simulink model "Phase_Estimator_4"  (R2020b)
settings: Solver=ode3  StartTime=0.0  StopTime=t(end)  FixedStep=1/60  RelTol=1e-3  EnableMultiTasking=on
undefined symbols (not defined in the file or in its folder): Activity, gamma_d, gamma_omg, x_initial, zeta
settings Model: Creator=wangf7  LastModifiedBy=chukw
settings DataIOCC: LimitDataPoints=on  SaveFormat=Array  ReturnWorkspaceOutputs=off
settings OptimizationCC: ExpressionDepthLimit=2147483647  LifeSpan=inf
settings DebuggingCC: UnderspecifiedInitializationDetection=Classic  MergeDetectMultiDrivingBlocksExec=none  SolverPrmCheckMsg=warning  StateNameClashWarn=warning  SFUnexpectedBacktrackingDiag=warning  SFNoUnconditionalDefaultTransitionDiag=warning  SFExecutionAtInitializationDiag=none  ArithmeticOperatorsInVariantConditions=warning
settings HardwareCC: ProdBitPerPointer=32  ProdBitPerSizeT=32  ProdBitPerPtrDiffT=32  ProdLargestAtomicFloat=None  ProdIntDivRoundTo=Undefined  ProdEndianess=Unspecified  ProdWordSize=32  ProdHWDeviceType=32-bit Generic
settings ModelReferenceCC: PropagateSignalLabelsOutOfModel=off
settings SFSimCC: SimUseLocalCustomCode=off  CustomCodeUndefinedFunction=UseInterfaceOnly
settings RTWCC: RTWUseLocalCustomCode=off
settings CodeAppCC: StateflowObjectComments=on
settings GRTTargetCC: TargetLangStandard=C89/C90 (ANSI)
settings ConfigComp: CovMetricSettings=dw  CovSaveCumulativeToWorkspaceVar=on  CovSaveSingleToWorkspaceVar=on  CovExternalEMLEnable=off
settings ConfigurationSet: Description=SimMechanics 2G

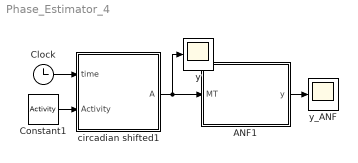
== system Phase_Estimator_4 ==
  ANF1 : Subsystem
  Clock : Clock
  Constant1 : Constant  Value=Activity
  circadian shifted1 : MATLAB Function  TreatAsAtomicUnit=on
  y : Scope
  y_ANF : Scope
  wires:
  circadian shifted1/1(A) -> y/1, ANF1/1(MT)
  Constant1/1 -> circadian shifted1/2(Activity)
  Clock/1 -> circadian shifted1/1(time)
  ANF1/1(y) -> y_ANF/1

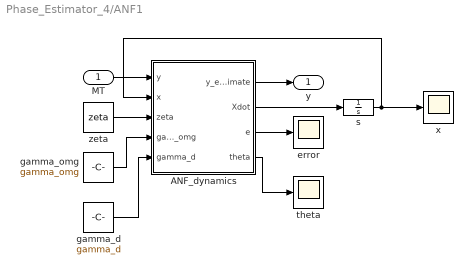
== system Phase_Estimator_4/ANF1 ==
  MT : Inport
  ANF_dynamics : MATLAB Function  TreatAsAtomicUnit=on
  error : Scope
  gamma_d : Constant  Value=gamma_d
  gamma_omg : Constant  Value=gamma_omg
  s : Integrator  InitialCondition=x_initial
  theta : Scope
  x : Scope
  zeta : Constant  Value=zeta
  y : Outport
  wires:
  MT/1 -> ANF_dynamics/1(y)
  s/1 -> x/1, ANF_dynamics/2(x)
  ANF_dynamics/2(Xdot) -> s/1
  ANF_dynamics/1(y_estimate) -> y/1
  ANF_dynamics/3(e) -> error/1
  ANF_dynamics/4(theta) -> theta/1
  zeta/1 -> ANF_dynamics/3(zeta)
  gamma_omg/1 -> ANF_dynamics/4(gamma_omg)
  gamma_d/1 -> ANF_dynamics/5(gamma_d)

== matlab function Phase_Estimator_4/circadian shifted1 ==
  data: time input; Activity input; A output
function A = fcn(time,Activity)
%#eml
A=interp1q(Activity(:,1),Activity(:,2),time);

== matlab function Phase_Estimator_4/ANF1/ANF_dynamics ==
  data: y_estimate output; y input; x input; Xdot output; e output; theta output; zeta input; gamma_omg input; gamma_d input
function [y_estimate,Xdot,e,theta] = fcn(y,x,zeta,gamma_omg,gamma_d)

x1 = x(1);%1st harmonic
x2 = x(2);%1st harmonic dot
x3 = x(3);%2nd harmonic
x4 = x(4);%2nd harmonic dot
x5 = x(5);%3rd harmonic
x6 = x(6);%3rd harmonic dot
x7 = x(7);%4th harmonic
x8 = x(8);%4th harmonic dot
dc = x(9);%dc
omg = 2*pi/24;%x(10);%omega

y_estimate = dc + 2*zeta/omg*x2  + zeta/omg*x4 + 2*zeta/omg/3*x6 + 2*zeta/omg/4*x8;
e = y - y_estimate;
if isnan(y)
    e=0;
end

Xdot = zeros(10,1);

Xdot(1,1) = x2;
Xdot(2,1) = omg^2*(e-x1);
Xdot(3,1) = x4;
Xdot(4,1) = (2*omg)^2*(e-x3);
Xdot(5,1) = x6;
Xdot(6,1) = (3*omg)^2*(e-x5);
Xdot(7,1) = x8;
Xdot(8,1) = (4*omg)^2*(e-x7);
Xdot(9,1) = gamma_d*e;
Xdot(10,1) = gamma_omg*(-x1*omg^2)*e;

theta=mod(-atan2(x(2),x(10)*x(1))+pi/2,2*pi);
